simulink model "orbit_process_noise"  (R2023b)
settings: Solver=VariableStepAuto  StartTime=0.0  StopTime=10.0  FixedStep=0.01  RelTol=1e-3
settings Model: Creator=plane  LastModifiedBy=plane

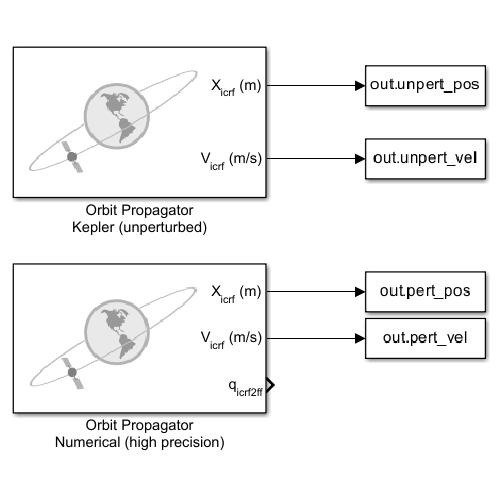
[thumbnail: Simulink's stored preview of the top-level diagram]
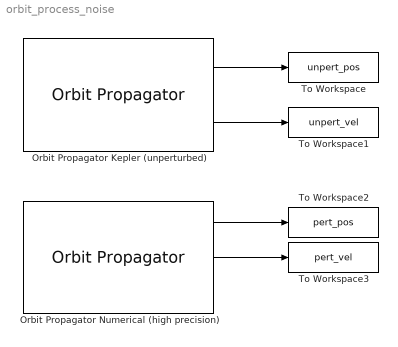
== system orbit_process_noise ==
  Orbit Propagator Kepler (unperturbed) : OrbitPropagator  dateOut=off  semiMajorAxis=orbit_param.semi_major  eccentricity=orbit_param.eccen  inclination=orbit_param.inclin_deg  raan=orbit_param.raan_deg  argPeriapsis=orbit_param.arg_periapse_deg  trueAnomaly=orbit_param.true_anom_deg  inertialPosition=[3649700.0 3308200.0 -4676600.0]  inertialVelocity=[-2750.8 6666.4 2573.4]  fixedPosition=[-4142689.0 -2676864.7 -4669861.6]  fixedVelocity=[1452.7 -6720.7 2568.1]  customR=3396200  customMu=4.305e13  customJ2=1.0826269e-03  customOmega=4.06125949e-3
  Orbit Propagator Numerical (high precision) : OrbitPropagator  propagator=Numerical (high precision)  dateOut=off  semiMajorAxis=orbit_param.semi_major  eccentricity=orbit_param.eccen  inclination=orbit_param.inclin_deg  raan=orbit_param.raan_deg  argPeriapsis=orbit_param.arg_periapse_deg  trueAnomaly=orbit_param.true_anom_deg  inertialPosition=[3649700.0 3308200.0 -4676600.0]  inertialVelocity=[-2750.8 6666.4 2573.4]  fixedPosition=[-4142689.0 -2676864.7 -4669861.6]  fixedVelocity=[1452.7 -6720.7 2568.1]  customR=3396200  customMu=4.305e13  customJ2=1.0826269e-03  customOmega=4.06125949e-3  outputTransform=on
  To Workspace : ToWorkspace  VariableName=unpert_pos  SaveFormat=Timeseries  SampleTime=-1
  To Workspace1 : ToWorkspace  VariableName=unpert_vel  SaveFormat=Timeseries  SampleTime=-1
  To Workspace2 : ToWorkspace  VariableName=pert_pos  SaveFormat=Timeseries  SampleTime=-1
  To Workspace3 : ToWorkspace  VariableName=pert_vel  SaveFormat=Timeseries  SampleTime=-1
  wires:
  Orbit Propagator Kepler (unperturbed)/1 -> To Workspace/1
  Orbit Propagator Kepler (unperturbed)/2 -> To Workspace1/1
  Orbit Propagator Numerical (high precision)/1 -> To Workspace2/1
  Orbit Propagator Numerical (high precision)/2 -> To Workspace3/1
